simulink model "warplab_mimo_4x4"  (Simulink 6.5)
settings: Solver=ode45  StartTime=0.0  StopTime=20000  RelTol=1e-3
undefined symbols (not defined in the file): gcbh, xlBlockLoadCallback
libraries: xbsIndex_r4 x188
(part 14 of 17)

== system warplab_mimo_4x4/Radio_3_Inputs/ADC_I ==
  Constant1 : Constant  Value=0  OutDataType=sfix(16)  ConRadixGroup=Use specified scaling  OutScaling=2^0  SampleTime=inf  FramePeriod=inf
  Radio_3_ADC_I : Subsystem  mask{adc_sample_period=1}
      mask prompts: adc_sample_period "Sample Period"
      mask Display: image(imread('WARP_Logo.jpg'))
  Register : S-Function  LoadFcn=xlBlockLoadCallback(gcbh);  FunctionName=sysgen  Parameters=ptable_  mask(Xilinx Register Block){init=0, rst_sgadvanced=, rst=off, en_sgadvanced=, en=off, dbl_ovrd_sgadvanced=, dbl_ovrd=off, xl_use_area_sgadvanced=, xl_use_area=off, xl_area=[0,0,0,0,0,0,0], has_advanced_control=0, sggui_pos=-1,-1,-1,-1, block_type=register, block_version=8.2, sg_icon_stat=35,28,1,1,white,blue,0,ac6b57db, sg_mask_display=|, sg_list_contents=, sg_blockgui_xml=}
      mask sg_mask_display=|
      | fprintf('','COMMENT: begin icon graphics');
      | patch([0 35 35 0 ],[0 0 28 28 ],[0.77 0.82 0.91]);
      | patch([10 5 12 5 10 17 19 21 29 23 17 13 21 13 17 23 29 21 19 17 10 ],[3 8 15 22 27 27 25 27 27 21 27 23 15 7 3 9 3 3 5 3 3 ],[0.98 0.96 0.92]);
      | plot([0 0 35 35 0 ],[0 28 28 0 0 ]);
      | fprintf('','COMMENT: end icon graphics');
      | fprintf('','COMMENT: begin icon text');
      | color('black');port_label('input',1,'d');
      | color('black');port_label('output',1,'q');
      | color('black');disp('\bf{z^{-1}}','texmode','on');
      | fprintf('','COMMENT: end icon text');
      mask prompts: init "Initial value"; rst_sgadvanced ""; rst "Provide synchronous reset port"; en_sgadvanced ""; en "Provide enable port"; dbl_ovrd_sgadvanced ""; dbl_ovrd "Override with doubles"; xl_use_area_sgadvanced ""; xl_use_area "Define FPGA area for resource estimation"; xl_area "FPGA area [slices, FFs, BRAMs, LUTs, IOBs, emb. mults, TBUFs]"; has_advanced_control ""; sggui_pos ""; block_type ""; block_version ""; sg_icon_stat ""; sg_mask_display ""; sg_list_contents ""; sg_blockgui_xml ""
      mask help: Xilinx Register
      mask init: same as warplab_mimo_4x4/Mem_Control/Register
      settings: CopyFcn=xlBlockMoveCallback(gcbh);  DeleteFcn=xlDestroyGui(gcbh);  ModelCloseFcn=xlDestroyGui(gcbh);  PreSaveFcn=xlBlockPreSaveCallback(gcbh);  PostSaveFcn=xlBlockPostSaveCallback(gcbh);  DestroyFcn=xlDestroyGui(gcbh);  OpenFcn=xlOpenGui(gcbh, 'register_gui.xml', @xlmagicenablement, -1)  CloseFcn=xlDestroyGui(gcbh);  MoveFcn=xlBlockMoveCallback(gcbh);
      mask Help: eval('xlWeb(xlhtmldoclink(''Register''))');
      mask Display:
      | fprintf('','COMMENT: begin icon graphics');
      | patch([0 35 35 0 ],[0 0 28 28 ],[0.77 0.82 0.91]);
      | patch([10 5 12 5 10 17 19 21 29 23 17 13 21 13 17 23 29 21 19 17 10 ],[3 8 15 22 27 27 25 27 27 21 27 23 15 7 3 9 3 3 5 3 3 ],[0.98 0.96 0.92]);
      | plot([0 0 35 35 0 ],[0 28 28 0 0 ]);
      | fprintf('','COMMENT: end icon graphics');
      | fprintf('','COMMENT: begin icon text');
      | color('black');port_label('input',1,'d');
      | color('black');port_label('output',1,'q');
      | color('black');disp('\bf{z^{-1}}','texmode','on');
      | fprintf('','COMMENT: end icon text');
  radio3_ADC_I_OTR : S-Function  LoadFcn=xlBlockLoadCallback(gcbh);  FunctionName=sysgen  Parameters=ptable_  mask(Xilinx Gateway In Block){infoedit=Gateway in block.  Converts inputs of type Simulink integer, double and fixed point to  Xilinx fixed point type.<P><P>Hardware notes:  In hardware these blocks become top level input ports., arith_type_sgadvanced=, arith_type=Unsigned, n_bits=1, bin_pt=0, quantization_sgadvanced=, quantization=Round  (unbiased: +/- Inf), overflow_sgadvanced=, overflow=Saturate, period=1, dbl_ovrd_sgadvanced=, dbl_ovrd=off, timing_constraint_sgadvanced=, timing_constraint=None, locs_specified_sgadvanced=, locs_specified=off, LOCs={}, xl_use_area_sgadvanced=, xl_use_area=off, xl_area=[0,0,0,0,0,0,0], sginterface=, has_advanced_control=0, sggui_pos=20,20,356,432, block_type=gatewayin, block_version=VER_STRING_GOES_HERE, sg_icon_stat=55,12,1,1,white,yellow,0,4bb76ffd, sg_mask_display=|, sg_list_contents=, sg_blockgui_xml=}
      mask sg_mask_display=|
      | fprintf('','COMMENT: begin icon graphics ');
      | patch([0 55 55 0 ],[0 0 12 12 ],[0.95 0.93 0.65]);
      | patch([24 22 25 22 24 27 28 29 32 29 26 24 27 24 26 29 32 29 28 27 24 ],[1 3 6 9 11 11 10 11 11 8 11 9 6 3 1 4 1 1 2 1 1 ],[0.98 0.96 0.92]);
      | plot([0 0 55 55 0 ],[0 12 12 0 0 ]);
      | fprintf('','COMMENT: end icon graphics');
      |
      | fprintf('','COMMENT: begin icon text ');
      | color('black');port_label('input',1,'\fontsize{11pt}\bf In ','texmode','on');
      | color('black');port_label('output',1,' ');
      | fprintf('','COMMENT: end icon text');
      | fprintf('','COMMENT: Make no changes above this line -- machine generated code. ');
      mask prompts: infoedit ""; arith_type_sgadvanced ""; arith_type "Output type"; n_bits "Number of bits"; bin_pt "Binary point"; quantization_sgadvanced ""; overflow_sgadvanced ""; period "Sample period"; dbl_ovrd_sgadvanced ""; dbl_ovrd "Override with doubles"; timing_constraint_sgadvanced ""; timing_constraint "IOB timing constraint"; locs_specified_sgadvanced ""; locs_specified "Specify IOB location constraints"; LOCs "IOB pad locations (specify as cell array {'MSB', ..., 'LSB'})"; xl_use_area_sgadvanced ""; xl_use_area "Define FPGA area for resource estimation"; xl_area "FPGA area [slices, FFs, BRAMs, LUTs, IOBs, emb. mults, TBUFs]"; sginterface ""; has_advanced_control ""; sggui_pos ""; block_type ""; block_version ""; sg_icon_stat ""; sg_mask_display ""; sg_list_contents ""; sg_blockgui_xml ""
      mask help:
      | Gateway in block.  Converts inputs of type Simulink integer, double and fixed point to  Xilinx fixed point type.
      |
      | Hardware notes:  In hardware these blocks become top level input ports.
      mask init: same as warplab_mimo_4x4/StartCapture
      settings: CopyFcn=xlBlockMoveCallback(gcbh);  DeleteFcn=xlDestroyGui(gcbh);  ModelCloseFcn=xlDestroyGui(gcbh);  PreSaveFcn=xlBlockPreSaveCallback(gcbh);  PostSaveFcn=xlBlockPostSaveCallback(gcbh);  DestroyFcn=xlDestroyGui(gcbh);  OpenFcn=xlOpenGui(gcbh, 'gatewayin_gui.xml', @gatewayinenablement, @gatewayinaction)  CloseFcn=xlDestroyGui(gcbh);  MoveFcn=xlBlockMoveCallback(gcbh);
      mask Help: eval('xlWeb(xlhtmldoclink(''Gateway In''))');
      mask StyleString: edit,edit,popup(Boolean|Signed  (2's comp)|Unsigned),edit,edit,edit,popup(Truncate|Round  (unbiased: +/- Inf)),edit,popup(Wrap|Saturate|Flag as error),edit,edit,checkbox,edit,popup(None|Data Rate),edit,checkbox,edit,edit,checkbox,edit,edit,edit,edit,edit,edit,edit,edit,edit,edit
      mask Display:
      | fprintf('','COMMENT: begin icon graphics ');
      | patch([0 55 55 0 ],[0 0 12 12 ],[0.95 0.93 0.65]);
      | patch([24 22 25 22 24 27 28 29 32 29 26 24 27 24 26 29 32 29 28 27 24 ],[1 3 6 9 11 11 10 11 11 8 11 9 6 3 1 4 1 1 2 1 1 ],[0.98 0.96 0.92]);
      | plot([0 0 55 55 0 ],[0 12 12 0 0 ]);
      | fprintf('','COMMENT: end icon graphics');
      | 
      | fprintf('','COMMENT: begin icon text ');
      | color('black');port_label('input',1,'\fontsize{11pt}\bf In ','texmode','on');
      | color('black');port_label('output',1,' ');
      | fprintf('','COMMENT: end icon text');
      | fprintf('','COMMENT: Make no changes above this line -- machine generated code. ');
  OTR I : Outport
  ADC I : Outport  Port=2
  wires:
  Register/1 -> ADC I/1
  radio3_ADC_I_OTR/1 -> OTR I/1
  Radio_3_ADC_I/1(I_out) -> Register/1
  Constant1/1 -> radio3_ADC_I_OTR/1, Radio_3_ADC_I/1(I)

== system warplab_mimo_4x4/Radio_3_Inputs/ADC_Q ==
  Constant1 : Constant  Value=0  OutDataType=sfix(16)  ConRadixGroup=Use specified scaling  OutScaling=2^0  SampleTime=inf  FramePeriod=inf
  Radio_3_ADC_Q : Subsystem  mask{adc_sample_period=1}
      mask Display: image(imread('WARP_Logo.jpg'))
  Register : S-Function  LoadFcn=xlBlockLoadCallback(gcbh);  FunctionName=sysgen  Parameters=ptable_  mask(Xilinx Register Block){init=0, rst_sgadvanced=, rst=off, en_sgadvanced=, en=off, dbl_ovrd_sgadvanced=, dbl_ovrd=off, xl_use_area_sgadvanced=, xl_use_area=off, xl_area=[0,0,0,0,0,0,0], has_advanced_control=0, sggui_pos=-1,-1,-1,-1, block_type=register, block_version=8.2, sg_icon_stat=35,28,1,1,white,blue,0,ac6b57db, sg_mask_display=|, sg_list_contents=, sg_blockgui_xml=}
      mask sg_mask_display=|
      | fprintf('','COMMENT: begin icon graphics');
      | patch([0 35 35 0 ],[0 0 28 28 ],[0.77 0.82 0.91]);
      | patch([10 5 12 5 10 17 19 21 29 23 17 13 21 13 17 23 29 21 19 17 10 ],[3 8 15 22 27 27 25 27 27 21 27 23 15 7 3 9 3 3 5 3 3 ],[0.98 0.96 0.92]);
      | plot([0 0 35 35 0 ],[0 28 28 0 0 ]);
      | fprintf('','COMMENT: end icon graphics');
      | fprintf('','COMMENT: begin icon text');
      | color('black');port_label('input',1,'d');
      | color('black');port_label('output',1,'q');
      | color('black');disp('\bf{z^{-1}}','texmode','on');
      | fprintf('','COMMENT: end icon text');
      mask prompts: init "Initial value"; rst_sgadvanced ""; rst "Provide synchronous reset port"; en_sgadvanced ""; en "Provide enable port"; dbl_ovrd_sgadvanced ""; dbl_ovrd "Override with doubles"; xl_use_area_sgadvanced ""; xl_use_area "Define FPGA area for resource estimation"; xl_area "FPGA area [slices, FFs, BRAMs, LUTs, IOBs, emb. mults, TBUFs]"; has_advanced_control ""; sggui_pos ""; block_type ""; block_version ""; sg_icon_stat ""; sg_mask_display ""; sg_list_contents ""; sg_blockgui_xml ""
      mask help: Xilinx Register
      mask init: same as warplab_mimo_4x4/Mem_Control/Register
      settings: CopyFcn=xlBlockMoveCallback(gcbh);  DeleteFcn=xlDestroyGui(gcbh);  ModelCloseFcn=xlDestroyGui(gcbh);  PreSaveFcn=xlBlockPreSaveCallback(gcbh);  PostSaveFcn=xlBlockPostSaveCallback(gcbh);  DestroyFcn=xlDestroyGui(gcbh);  OpenFcn=xlOpenGui(gcbh, 'register_gui.xml', @xlmagicenablement, -1)  CloseFcn=xlDestroyGui(gcbh);  MoveFcn=xlBlockMoveCallback(gcbh);
      mask Help: eval('xlWeb(xlhtmldoclink(''Register''))');
      mask Display:
      | fprintf('','COMMENT: begin icon graphics');
      | patch([0 35 35 0 ],[0 0 28 28 ],[0.77 0.82 0.91]);
      | patch([10 5 12 5 10 17 19 21 29 23 17 13 21 13 17 23 29 21 19 17 10 ],[3 8 15 22 27 27 25 27 27 21 27 23 15 7 3 9 3 3 5 3 3 ],[0.98 0.96 0.92]);
      | plot([0 0 35 35 0 ],[0 28 28 0 0 ]);
      | fprintf('','COMMENT: end icon graphics');
      | fprintf('','COMMENT: begin icon text');
      | color('black');port_label('input',1,'d');
      | color('black');port_label('output',1,'q');
      | color('black');disp('\bf{z^{-1}}','texmode','on');
      | fprintf('','COMMENT: end icon text');
  radio3_ADC_Q_OTR : S-Function  LoadFcn=xlBlockLoadCallback(gcbh);  FunctionName=sysgen  Parameters=ptable_  mask(Xilinx Gateway In Block){infoedit=Gateway in block.  Converts inputs of type Simulink integer, double and fixed point to  Xilinx fixed point type.<P><P>Hardware notes:  In hardware these blocks become top level input ports., arith_type_sgadvanced=, arith_type=Unsigned, n_bits=1, bin_pt=0, quantization_sgadvanced=, quantization=Round  (unbiased: +/- Inf), overflow_sgadvanced=, overflow=Saturate, period=1, dbl_ovrd_sgadvanced=, dbl_ovrd=off, timing_constraint_sgadvanced=, timing_constraint=None, locs_specified_sgadvanced=, locs_specified=off, LOCs={}, xl_use_area_sgadvanced=, xl_use_area=off, xl_area=[0,0,0,0,0,0,0], sginterface=, has_advanced_control=0, sggui_pos=20,20,356,432, block_type=gatewayin, block_version=VER_STRING_GOES_HERE, sg_icon_stat=55,12,1,1,white,yellow,0,4bb76ffd, sg_mask_display=|, sg_list_contents=, sg_blockgui_xml=}
      mask sg_mask_display=|
      | fprintf('','COMMENT: begin icon graphics ');
      | patch([0 55 55 0 ],[0 0 12 12 ],[0.95 0.93 0.65]);
      | patch([24 22 25 22 24 27 28 29 32 29 26 24 27 24 26 29 32 29 28 27 24 ],[1 3 6 9 11 11 10 11 11 8 11 9 6 3 1 4 1 1 2 1 1 ],[0.98 0.96 0.92]);
      | plot([0 0 55 55 0 ],[0 12 12 0 0 ]);
      | fprintf('','COMMENT: end icon graphics');
      |
      | fprintf('','COMMENT: begin icon text ');
      | color('black');port_label('input',1,'\fontsize{11pt}\bf In ','texmode','on');
      | color('black');port_label('output',1,' ');
      | fprintf('','COMMENT: end icon text');
      | fprintf('','COMMENT: Make no changes above this line -- machine generated code. ');
      mask prompts: infoedit ""; arith_type_sgadvanced ""; arith_type "Output type"; n_bits "Number of bits"; bin_pt "Binary point"; quantization_sgadvanced ""; overflow_sgadvanced ""; period "Sample period"; dbl_ovrd_sgadvanced ""; dbl_ovrd "Override with doubles"; timing_constraint_sgadvanced ""; timing_constraint "IOB timing constraint"; locs_specified_sgadvanced ""; locs_specified "Specify IOB location constraints"; LOCs "IOB pad locations (specify as cell array {'MSB', ..., 'LSB'})"; xl_use_area_sgadvanced ""; xl_use_area "Define FPGA area for resource estimation"; xl_area "FPGA area [slices, FFs, BRAMs, LUTs, IOBs, emb. mults, TBUFs]"; sginterface ""; has_advanced_control ""; sggui_pos ""; block_type ""; block_version ""; sg_icon_stat ""; sg_mask_display ""; sg_list_contents ""; sg_blockgui_xml ""
      mask help:
      | Gateway in block.  Converts inputs of type Simulink integer, double and fixed point to  Xilinx fixed point type.
      |
      | Hardware notes:  In hardware these blocks become top level input ports.
      mask init: same as warplab_mimo_4x4/StartCapture
      settings: CopyFcn=xlBlockMoveCallback(gcbh);  DeleteFcn=xlDestroyGui(gcbh);  ModelCloseFcn=xlDestroyGui(gcbh);  PreSaveFcn=xlBlockPreSaveCallback(gcbh);  PostSaveFcn=xlBlockPostSaveCallback(gcbh);  DestroyFcn=xlDestroyGui(gcbh);  OpenFcn=xlOpenGui(gcbh, 'gatewayin_gui.xml', @gatewayinenablement, @gatewayinaction)  CloseFcn=xlDestroyGui(gcbh);  MoveFcn=xlBlockMoveCallback(gcbh);
      mask Help: eval('xlWeb(xlhtmldoclink(''Gateway In''))');
      mask StyleString: edit,edit,popup(Boolean|Signed  (2's comp)|Unsigned),edit,edit,edit,popup(Truncate|Round  (unbiased: +/- Inf)),edit,popup(Wrap|Saturate|Flag as error),edit,edit,checkbox,edit,popup(None|Data Rate),edit,checkbox,edit,edit,checkbox,edit,edit,edit,edit,edit,edit,edit,edit,edit,edit
      mask Display:
      | fprintf('','COMMENT: begin icon graphics ');
      | patch([0 55 55 0 ],[0 0 12 12 ],[0.95 0.93 0.65]);
      | patch([24 22 25 22 24 27 28 29 32 29 26 24 27 24 26 29 32 29 28 27 24 ],[1 3 6 9 11 11 10 11 11 8 11 9 6 3 1 4 1 1 2 1 1 ],[0.98 0.96 0.92]);
      | plot([0 0 55 55 0 ],[0 12 12 0 0 ]);
      | fprintf('','COMMENT: end icon graphics');
      | 
      | fprintf('','COMMENT: begin icon text ');
      | color('black');port_label('input',1,'\fontsize{11pt}\bf In ','texmode','on');
      | color('black');port_label('output',1,' ');
      | fprintf('','COMMENT: end icon text');
      | fprintf('','COMMENT: Make no changes above this line -- machine generated code. ');
  OTR Q : Outport
  ADC Q : Outport  Port=2
  wires:
  Register/1 -> ADC Q/1
  Constant1/1 -> radio3_ADC_Q_OTR/1, Radio_3_ADC_Q/1(Q)
  Radio_3_ADC_Q/1(Q_out) -> Register/1
  radio3_ADC_Q_OTR/1 -> OTR Q/1

== system warplab_mimo_4x4/Radio_3_Inputs/Concatenates_1 ==
  OTR_I : Inport
  ADC_I : Inport  Port=2
  OTR_Q : Inport  Port=3
  ADC_Q : Inport  Port=4
  Concat1 : S-Function  LoadFcn=xlBlockLoadCallback(gcbh);  FunctionName=sysgen  Parameters=ptable_  mask(Xilinx Bus Concatenator Block){infoedit=Concatenates two or more inputs.  Output will be cast to an unsigned value with the binary point at zero., num_inputs=2, dbl_ovrd_sgadvanced=, dbl_ovrd=off, has_advanced_control=0, sggui_pos=-1,-1,-1,-1, block_type=concat, block_version=8.2, sg_icon_stat=30,38,2,1,white,blue,0,59d62d82, sg_mask_display=|, sg_list_contents=, sg_blockgui_xml=}
      mask sg_mask_display=|
      | fprintf('','COMMENT: begin icon graphics');
      | patch([0 30 30 0 ],[0 0 38 38 ],[0.77 0.82 0.91]);
      | patch([7 2 9 2 7 15 17 19 27 20 14 9 15 9 14 20 27 19 17 15 7 ],[7 12 19 26 31 31 29 31 31 24 30 25 19 13 8 14 7 7 9 7 7 ],[0.98 0.96 0.92]);
      | plot([0 0 30 30 0 ],[0 38 38 0 0 ]);
      | fprintf('','COMMENT: end icon graphics');
      | fprintf('','COMMENT: begin icon text');
      | color('black');port_label('input',1,'hi');
      | color('black');port_label('input',2,'lo');
      | fprintf('','COMMENT: end icon text');
      mask prompts: infoedit ""; num_inputs "Number of inputs"; dbl_ovrd_sgadvanced ""; dbl_ovrd "Override with doubles"; has_advanced_control ""; sggui_pos ""; block_type ""; block_version ""; sg_icon_stat ""; sg_mask_display ""; sg_list_contents ""; sg_blockgui_xml ""
      mask help: Concatenates two or more inputs. Output will be cast to an unsigned value with the binary point at zero.
      mask init: same as warplab_mimo_4x4/Radio_1_Inputs/Concatenates_1/Concat1
      settings: CopyFcn=xlBlockMoveCallback(gcbh);  DeleteFcn=xlDestroyGui(gcbh);  ModelCloseFcn=xlDestroyGui(gcbh);  PreSaveFcn=xlBlockPreSaveCallback(gcbh);  PostSaveFcn=xlBlockPostSaveCallback(gcbh);  DestroyFcn=xlDestroyGui(gcbh);  OpenFcn=xlOpenGui(gcbh, 'concat_gui.xml', @xlmagicenablement, -1)  CloseFcn=xlDestroyGui(gcbh);  MoveFcn=xlBlockMoveCallback(gcbh);
      mask Help: eval('xlWeb(xlhtmldoclink(''Concat''))');
      mask Display:
      | fprintf('','COMMENT: begin icon graphics');
      | patch([0 30 30 0 ],[0 0 38 38 ],[0.77 0.82 0.91]);
      | patch([7 2 9 2 7 15 17 19 27 20 14 9 15 9 14 20 27 19 17 15 7 ],[7 12 19 26 31 31 29 31 31 24 30 25 19 13 8 14 7 7 9 7 7 ],[0.98 0.96 0.92]);
      | plot([0 0 30 30 0 ],[0 38 38 0 0 ]);
      | fprintf('','COMMENT: end icon graphics');
      | fprintf('','COMMENT: begin icon text');
      | color('black');port_label('input',1,'hi');
      | color('black');port_label('input',2,'lo');
      | fprintf('','COMMENT: end icon text');
  Concat2 : S-Function  LoadFcn=xlBlockLoadCallback(gcbh);  FunctionName=sysgen  Parameters=ptable_  mask(Xilinx Bus Concatenator Block){infoedit=Concatenates two or more inputs.  Output will be cast to an unsigned value with the binary point at zero., num_inputs=2, dbl_ovrd_sgadvanced=, dbl_ovrd=off, has_advanced_control=0, sggui_pos=-1,-1,-1,-1, block_type=concat, block_version=8.2, sg_icon_stat=30,38,2,1,white,blue,0,59d62d82, sg_mask_display=|, sg_list_contents=, sg_blockgui_xml=}
      mask sg_mask_display=|
      | fprintf('','COMMENT: begin icon graphics');
      | patch([0 30 30 0 ],[0 0 38 38 ],[0.77 0.82 0.91]);
      | patch([7 2 9 2 7 15 17 19 27 20 14 9 15 9 14 20 27 19 17 15 7 ],[7 12 19 26 31 31 29 31 31 24 30 25 19 13 8 14 7 7 9 7 7 ],[0.98 0.96 0.92]);
      | plot([0 0 30 30 0 ],[0 38 38 0 0 ]);
      | fprintf('','COMMENT: end icon graphics');
      | fprintf('','COMMENT: begin icon text');
      | color('black');port_label('input',1,'hi');
      | color('black');port_label('input',2,'lo');
      | fprintf('','COMMENT: end icon text');
      mask prompts: infoedit ""; num_inputs "Number of inputs"; dbl_ovrd_sgadvanced ""; dbl_ovrd "Override with doubles"; has_advanced_control ""; sggui_pos ""; block_type ""; block_version ""; sg_icon_stat ""; sg_mask_display ""; sg_list_contents ""; sg_blockgui_xml ""
      mask help: Concatenates two or more inputs. Output will be cast to an unsigned value with the binary point at zero.
      mask init: same as warplab_mimo_4x4/Radio_1_Inputs/Concatenates_1/Concat1
      settings: CopyFcn=xlBlockMoveCallback(gcbh);  DeleteFcn=xlDestroyGui(gcbh);  ModelCloseFcn=xlDestroyGui(gcbh);  PreSaveFcn=xlBlockPreSaveCallback(gcbh);  PostSaveFcn=xlBlockPostSaveCallback(gcbh);  DestroyFcn=xlDestroyGui(gcbh);  OpenFcn=xlOpenGui(gcbh, 'concat_gui.xml', @xlmagicenablement, -1)  CloseFcn=xlDestroyGui(gcbh);  MoveFcn=xlBlockMoveCallback(gcbh);
      mask Help: eval('xlWeb(xlhtmldoclink(''Concat''))');
      mask Display:
      | fprintf('','COMMENT: begin icon graphics');
      | patch([0 30 30 0 ],[0 0 38 38 ],[0.77 0.82 0.91]);
      | patch([7 2 9 2 7 15 17 19 27 20 14 9 15 9 14 20 27 19 17 15 7 ],[7 12 19 26 31 31 29 31 31 24 30 25 19 13 8 14 7 7 9 7 7 ],[0.98 0.96 0.92]);
      | plot([0 0 30 30 0 ],[0 38 38 0 0 ]);
      | fprintf('','COMMENT: end icon graphics');
      | fprintf('','COMMENT: begin icon text');
      | color('black');port_label('input',1,'hi');
      | color('black');port_label('input',2,'lo');
      | fprintf('','COMMENT: end icon text');
  Concat3 : S-Function  LoadFcn=xlBlockLoadCallback(gcbh);  FunctionName=sysgen  Parameters=ptable_  mask(Xilinx Bus Concatenator Block){infoedit=Concatenates two or more inputs.  Output will be cast to an unsigned value with the binary point at zero., num_inputs=2, dbl_ovrd_sgadvanced=, dbl_ovrd=off, has_advanced_control=0, sggui_pos=-1,-1,-1,-1, block_type=concat, block_version=8.2, sg_icon_stat=25,80,2,1,white,blue,0,59d62d82, sg_mask_display=|, sg_list_contents=, sg_blockgui_xml=}
      mask sg_mask_display=|
      | fprintf('','COMMENT: begin icon graphics');
      | patch([0 25 25 0 ],[0 0 80 80 ],[0.77 0.82 0.91]);
      | patch([6 2 8 2 6 13 15 17 24 18 13 9 14 9 13 18 24 17 15 13 6 ],[30 34 40 46 50 50 48 50 50 44 49 45 40 35 31 36 30 30 32 30 30 ],[0.98 0.96 0.92]);
      | plot([0 0 25 25 0 ],[0 80 80 0 0 ]);
      | fprintf('','COMMENT: end icon graphics');
      | fprintf('','COMMENT: begin icon text');
      | color('black');port_label('input',1,'hi');
      | color('black');port_label('input',2,'lo');
      | fprintf('','COMMENT: end icon text');
      mask prompts: infoedit ""; num_inputs "Number of inputs"; dbl_ovrd_sgadvanced ""; dbl_ovrd "Override with doubles"; has_advanced_control ""; sggui_pos ""; block_type ""; block_version ""; sg_icon_stat ""; sg_mask_display ""; sg_list_contents ""; sg_blockgui_xml ""
      mask help: Concatenates two or more inputs. Output will be cast to an unsigned value with the binary point at zero.
      mask init: same as warplab_mimo_4x4/Radio_1_Inputs/Concatenates_1/Concat1
      settings: CopyFcn=xlBlockMoveCallback(gcbh);  DeleteFcn=xlDestroyGui(gcbh);  ModelCloseFcn=xlDestroyGui(gcbh);  PreSaveFcn=xlBlockPreSaveCallback(gcbh);  PostSaveFcn=xlBlockPostSaveCallback(gcbh);  DestroyFcn=xlDestroyGui(gcbh);  OpenFcn=xlOpenGui(gcbh, 'concat_gui.xml', @xlmagicenablement, -1)  CloseFcn=xlDestroyGui(gcbh);  MoveFcn=xlBlockMoveCallback(gcbh);
      mask Help: eval('xlWeb(xlhtmldoclink(''Concat''))');
      mask Display:
      | fprintf('','COMMENT: begin icon graphics');
      | patch([0 25 25 0 ],[0 0 80 80 ],[0.77 0.82 0.91]);
      | patch([6 2 8 2 6 13 15 17 24 18 13 9 14 9 13 18 24 17 15 13 6 ],[30 34 40 46 50 50 48 50 50 44 49 45 40 35 31 36 30 30 32 30 30 ],[0.98 0.96 0.92]);
      | plot([0 0 25 25 0 ],[0 80 80 0 0 ]);
      | fprintf('','COMMENT: end icon graphics');
      | fprintf('','COMMENT: begin icon text');
      | color('black');port_label('input',1,'hi');
      | color('black');port_label('input',2,'lo');
      | fprintf('','COMMENT: end icon text');
  Concat4 : S-Function  LoadFcn=xlBlockLoadCallback(gcbh);  FunctionName=sysgen  Parameters=ptable_  mask(Xilinx Bus Concatenator Block){infoedit=Concatenates two or more inputs.  Output will be cast to an unsigned value with the binary point at zero., num_inputs=2, dbl_ovrd_sgadvanced=, dbl_ovrd=off, has_advanced_control=0, sggui_pos=-1,-1,-1,-1, block_type=concat, block_version=8.2, sg_icon_stat=25,80,2,1,white,blue,0,59d62d82, sg_mask_display=|, sg_list_contents=, sg_blockgui_xml=}
      mask sg_mask_display=|
      | fprintf('','COMMENT: begin icon graphics');
      | patch([0 25 25 0 ],[0 0 80 80 ],[0.77 0.82 0.91]);
      | patch([6 2 8 2 6 13 15 17 24 18 13 9 14 9 13 18 24 17 15 13 6 ],[30 34 40 46 50 50 48 50 50 44 49 45 40 35 31 36 30 30 32 30 30 ],[0.98 0.96 0.92]);
      | plot([0 0 25 25 0 ],[0 80 80 0 0 ]);
      | fprintf('','COMMENT: end icon graphics');
      | fprintf('','COMMENT: begin icon text');
      | color('black');port_label('input',1,'hi');
      | color('black');port_label('input',2,'lo');
      | fprintf('','COMMENT: end icon text');
      mask prompts: infoedit ""; num_inputs "Number of inputs"; dbl_ovrd_sgadvanced ""; dbl_ovrd "Override with doubles"; has_advanced_control ""; sggui_pos ""; block_type ""; block_version ""; sg_icon_stat ""; sg_mask_display ""; sg_list_contents ""; sg_blockgui_xml ""
      mask help: Concatenates two or more inputs. Output will be cast to an unsigned value with the binary point at zero.
      mask init: same as warplab_mimo_4x4/Radio_1_Inputs/Concatenates_1/Concat1
      settings: CopyFcn=xlBlockMoveCallback(gcbh);  DeleteFcn=xlDestroyGui(gcbh);  ModelCloseFcn=xlDestroyGui(gcbh);  PreSaveFcn=xlBlockPreSaveCallback(gcbh);  PostSaveFcn=xlBlockPostSaveCallback(gcbh);  DestroyFcn=xlDestroyGui(gcbh);  OpenFcn=xlOpenGui(gcbh, 'concat_gui.xml', @xlmagicenablement, -1)  CloseFcn=xlDestroyGui(gcbh);  MoveFcn=xlBlockMoveCallback(gcbh);
      mask Help: eval('xlWeb(xlhtmldoclink(''Concat''))');
      mask Display:
      | fprintf('','COMMENT: begin icon graphics');
      | patch([0 25 25 0 ],[0 0 80 80 ],[0.77 0.82 0.91]);
      | patch([6 2 8 2 6 13 15 17 24 18 13 9 14 9 13 18 24 17 15 13 6 ],[30 34 40 46 50 50 48 50 50 44 49 45 40 35 31 36 30 30 32 30 30 ],[0.98 0.96 0.92]);
      | plot([0 0 25 25 0 ],[0 80 80 0 0 ]);
      | fprintf('','COMMENT: end icon graphics');
      | fprintf('','COMMENT: begin icon text');
      | color('black');port_label('input',1,'hi');
      | color('black');port_label('input',2,'lo');
      | fprintf('','COMMENT: end icon text');
  Concat5 : S-Function  LoadFcn=xlBlockLoadCallback(gcbh);  FunctionName=sysgen  Parameters=ptable_  mask(Xilinx Bus Concatenator Block){infoedit=Concatenates two or more inputs.  Output will be cast to an unsigned value with the binary point at zero., num_inputs=2, dbl_ovrd_sgadvanced=, dbl_ovrd=off, has_advanced_control=0, sggui_pos=-1,-1,-1,-1, block_type=concat, block_version=8.2, sg_icon_stat=25,80,2,1,white,blue,0,59d62d82, sg_mask_display=|, sg_list_contents=, sg_blockgui_xml=}
      mask sg_mask_display=|
      | fprintf('','COMMENT: begin icon graphics');
      | patch([0 25 25 0 ],[0 0 80 80 ],[0.77 0.82 0.91]);
      | patch([6 2 8 2 6 13 15 17 24 18 13 9 14 9 13 18 24 17 15 13 6 ],[30 34 40 46 50 50 48 50 50 44 49 45 40 35 31 36 30 30 32 30 30 ],[0.98 0.96 0.92]);
      | plot([0 0 25 25 0 ],[0 80 80 0 0 ]);
      | fprintf('','COMMENT: end icon graphics');
      | fprintf('','COMMENT: begin icon text');
      | color('black');port_label('input',1,'hi');
      | color('black');port_label('input',2,'lo');
      | fprintf('','COMMENT: end icon text');
      mask prompts: infoedit ""; num_inputs "Number of inputs"; dbl_ovrd_sgadvanced ""; dbl_ovrd "Override with doubles"; has_advanced_control ""; sggui_pos ""; block_type ""; block_version ""; sg_icon_stat ""; sg_mask_display ""; sg_list_contents ""; sg_blockgui_xml ""
      mask help: Concatenates two or more inputs. Output will be cast to an unsigned value with the binary point at zero.
      mask init: same as warplab_mimo_4x4/Radio_1_Inputs/Concatenates_1/Concat1
      settings: CopyFcn=xlBlockMoveCallback(gcbh);  DeleteFcn=xlDestroyGui(gcbh);  ModelCloseFcn=xlDestroyGui(gcbh);  PreSaveFcn=xlBlockPreSaveCallback(gcbh);  PostSaveFcn=xlBlockPostSaveCallback(gcbh);  DestroyFcn=xlDestroyGui(gcbh);  OpenFcn=xlOpenGui(gcbh, 'concat_gui.xml', @xlmagicenablement, -1)  CloseFcn=xlDestroyGui(gcbh);  MoveFcn=xlBlockMoveCallback(gcbh);
      mask Help: eval('xlWeb(xlhtmldoclink(''Concat''))');
      mask Display:
      | fprintf('','COMMENT: begin icon graphics');
      | patch([0 25 25 0 ],[0 0 80 80 ],[0.77 0.82 0.91]);
      | patch([6 2 8 2 6 13 15 17 24 18 13 9 14 9 13 18 24 17 15 13 6 ],[30 34 40 46 50 50 48 50 50 44 49 45 40 35 31 36 30 30 32 30 30 ],[0.98 0.96 0.92]);
      | plot([0 0 25 25 0 ],[0 80 80 0 0 ]);
      | fprintf('','COMMENT: end icon graphics');
      | fprintf('','COMMENT: begin icon text');
      | color('black');port_label('input',1,'hi');
      | color('black');port_label('input',2,'lo');
      | fprintf('','COMMENT: end icon text');
  Reinterpret : S-Function  LoadFcn=xlBlockLoadCallback(gcbh);  FunctionName=sysgen  Parameters=ptable_  mask(Xilinx Type Reinterpreter Block){infoedit=Changes signal type without altering the binary representation.   You can changed the signal between signed and unsigned, and relocate the binary point.<P><P>Hardware notes: In hardware this block costs nothing.<P><P>Example:  Suppose the input is 6 bits wide, signed, with 2 fractional bits, and the output is forced to unsigned with 0 fractional bits.  Then an input of -2.0 (1110.00 in binary 2's complement) becomes an output of 56 (111000 in binary)., force_arith_type_sgadvanced=, force_arith_type=on, arith_type_sgadvanced=, arith_type=Unsigned, force_bin_pt_sgadvanced=, force_bin_pt=on, bin_pt=0, has_advanced_control=0, sggui_pos=20,20,356,309, block_type=reinterpret, block_version=8.2, sg_icon_stat=35,20,1,1,white,blue,0,8982c1db, sg_mask_display=|, sg_list_contents=, sg_blockgui_xml=}
      mask sg_mask_display=|
      | fprintf('','COMMENT: begin icon graphics');
      | patch([0 35 35 0 ],[0 0 20 20 ],[0.77 0.82 0.91]);
      | patch([12 9 14 9 12 17 18 19 25 21 17 14 19 14 17 21 25 19 18 17 12 ],[2 5 10 15 18 18 17 18 18 14 18 15 10 5 2 6 2 2 3 2 2 ],[0.98 0.96 0.92]);
      | plot([0 0 35 35 0 ],[0 20 20 0 0 ]);
      | fprintf('','COMMENT: end icon graphics');
      | fprintf('','COMMENT: begin icon text');
      | color('black');disp('reinterpret');
      | fprintf('','COMMENT: end icon text');
      mask prompts: infoedit ""; force_arith_type_sgadvanced ""; force_arith_type "Force Arithmetic Type"; arith_type_sgadvanced ""; arith_type "Output Arithmetic Type"; force_bin_pt_sgadvanced ""; force_bin_pt "Force Binary Point"; bin_pt "Output Binary Point"; has_advanced_control ""; sggui_pos ""; block_type ""; block_version ""; sg_icon_stat ""; sg_mask_display ""; sg_list_contents ""; sg_blockgui_xml ""
      mask help:
      | Changes signal type without altering the binary representation.   You can changed the signal between signed and unsigned, and relocate the binary point.
      |
      | Hardware notes: In hardware this block costs nothing.
      |
      | Example:  Suppose the input is 6 bits wide, signed, with 2 fractional bits, and the output is forced to unsigned with 0 fractional bits.  Then an input of -2.0 (1110.00 in binary 2's complement) becomes an output of 56 (111000 in binary).
      mask init: same as warplab_mimo_4x4/Radio_1_Outputs/Reinterpret
      settings: CopyFcn=xlBlockMoveCallback(gcbh);  DeleteFcn=xlDestroyGui(gcbh);  ModelCloseFcn=xlDestroyGui(gcbh);  PreSaveFcn=xlBlockPreSaveCallback(gcbh);  PostSaveFcn=xlBlockPostSaveCallback(gcbh);  DestroyFcn=xlDestroyGui(gcbh);  OpenFcn=xlOpenGui(gcbh, 'reinterpret_gui.xml', @reinterpretenablement, -1)  CloseFcn=xlDestroyGui(gcbh);  MoveFcn=xlBlockMoveCallback(gcbh);
      mask Help: eval('xlWeb(xlhtmldoclink(''Reinterpret''))');
      mask StyleString: edit,edit,checkbox,edit,popup(Unsigned|Signed  (2's comp)),edit,checkbox,edit,edit,edit,edit,edit,edit,edit,edit,edit
      mask Display:
      | fprintf('','COMMENT: begin icon graphics');
      | patch([0 35 35 0 ],[0 0 20 20 ],[0.77 0.82 0.91]);
      | patch([12 9 14 9 12 17 18 19 25 21 17 14 19 14 17 21 25 19 18 17 12 ],[2 5 10 15 18 18 17 18 18 14 18 15 10 5 2 6 2 2 3 2 2 ],[0.98 0.96 0.92]);
      | plot([0 0 35 35 0 ],[0 20 20 0 0 ]);
      | fprintf('','COMMENT: end icon graphics');
      | fprintf('','COMMENT: begin icon text');
      | color('black');disp('reinterpret');
      | fprintf('','COMMENT: end icon text');
  Reinterpret1 : S-Function  LoadFcn=xlBlockLoadCallback(gcbh);  FunctionName=sysgen  Parameters=ptable_  mask(Xilinx Type Reinterpreter Block){infoedit=Changes signal type without altering the binary representation.   You can changed the signal between signed and unsigned, and relocate the binary point.<P><P>Hardware notes: In hardware this block costs nothing.<P><P>Example:  Suppose the input is 6 bits wide, signed, with 2 fractional bits, and the output is forced to unsigned with 0 fractional bits.  Then an input of -2.0 (1110.00 in binary 2's complement) becomes an output of 56 (111000 in binary)., force_arith_type_sgadvanced=, force_arith_type=on, arith_type_sgadvanced=, arith_type=Unsigned, force_bin_pt_sgadvanced=, force_bin_pt=on, bin_pt=0, has_advanced_control=0, sggui_pos=20,20,356,309, block_type=reinterpret, block_version=8.2, sg_icon_stat=35,20,1,1,white,blue,0,8982c1db, sg_mask_display=|, sg_list_contents=, sg_blockgui_xml=}
      mask sg_mask_display=|
      | fprintf('','COMMENT: begin icon graphics');
      | patch([0 35 35 0 ],[0 0 20 20 ],[0.77 0.82 0.91]);
      | patch([12 9 14 9 12 17 18 19 25 21 17 14 19 14 17 21 25 19 18 17 12 ],[2 5 10 15 18 18 17 18 18 14 18 15 10 5 2 6 2 2 3 2 2 ],[0.98 0.96 0.92]);
      | plot([0 0 35 35 0 ],[0 20 20 0 0 ]);
      | fprintf('','COMMENT: end icon graphics');
      | fprintf('','COMMENT: begin icon text');
      | color('black');disp('reinterpret');
      | fprintf('','COMMENT: end icon text');
      mask prompts: infoedit ""; force_arith_type_sgadvanced ""; force_arith_type "Force Arithmetic Type"; arith_type_sgadvanced ""; arith_type "Output Arithmetic Type"; force_bin_pt_sgadvanced ""; force_bin_pt "Force Binary Point"; bin_pt "Output Binary Point"; has_advanced_control ""; sggui_pos ""; block_type ""; block_version ""; sg_icon_stat ""; sg_mask_display ""; sg_list_contents ""; sg_blockgui_xml ""
      mask help:
      | Changes signal type without altering the binary representation.   You can changed the signal between signed and unsigned, and relocate the binary point.
      |
      | Hardware notes: In hardware this block costs nothing.
      |
      | Example:  Suppose the input is 6 bits wide, signed, with 2 fractional bits, and the output is forced to unsigned with 0 fractional bits.  Then an input of -2.0 (1110.00 in binary 2's complement) becomes an output of 56 (111000 in binary).
      mask init: same as warplab_mimo_4x4/Radio_1_Outputs/Reinterpret
      settings: CopyFcn=xlBlockMoveCallback(gcbh);  DeleteFcn=xlDestroyGui(gcbh);  ModelCloseFcn=xlDestroyGui(gcbh);  PreSaveFcn=xlBlockPreSaveCallback(gcbh);  PostSaveFcn=xlBlockPostSaveCallback(gcbh);  DestroyFcn=xlDestroyGui(gcbh);  OpenFcn=xlOpenGui(gcbh, 'reinterpret_gui.xml', @reinterpretenablement, -1)  CloseFcn=xlDestroyGui(gcbh);  MoveFcn=xlBlockMoveCallback(gcbh);
      mask Help: eval('xlWeb(xlhtmldoclink(''Reinterpret''))');
      mask StyleString: edit,edit,checkbox,edit,popup(Unsigned|Signed  (2's comp)),edit,checkbox,edit,edit,edit,edit,edit,edit,edit,edit,edit
      mask Display:
      | fprintf('','COMMENT: begin icon graphics');
      | patch([0 35 35 0 ],[0 0 20 20 ],[0.77 0.82 0.91]);
      | patch([12 9 14 9 12 17 18 19 25 21 17 14 19 14 17 21 25 19 18 17 12 ],[2 5 10 15 18 18 17 18 18 14 18 15 10 5 2 6 2 2 3 2 2 ],[0.98 0.96 0.92]);
      | plot([0 0 35 35 0 ],[0 20 20 0 0 ]);
      | fprintf('','COMMENT: end icon graphics');
      | fprintf('','COMMENT: begin icon text');
      | color('black');disp('reinterpret');
      | fprintf('','COMMENT: end icon text');
  zero : S-Function  LoadFcn=xlBlockLoadCallback(gcbh);  FunctionName=sysgen  Parameters=ptable_  mask(Xilinx Constant Block Block){arith_type_sgadvanced=, arith_type=Unsigned, const=0, n_bits=1, bin_pt=0, explicit_period_sgadvanced=, explicit_period=off, period=1, dsp48_infoedit=The use of this block for DSP48 instructions is deprecated.  Please use the Opmode block., equ=P=C, opselect_sgadvanced=, opselect=C, inp2_sgadvanced=, inp2=PCIN>>17, opr_sgadvanced=, opr=+, inp1_sgadvanced=, inp1=P, carry_sgadvanced=, carry=CIN, dbl_ovrd_sgadvanced=, dbl_ovrd=off, has_advanced_control=0, sggui_pos=-1,-1,-1,-1, block_type=constant, block_version=VER_STRING_GOES_HERE, sg_icon_stat=20,18,0,1,white,blue,0,c7c04a0c, sg_mask_display=|, sg_list_contents=, sg_blockgui_xml=}
      mask sg_mask_display=|
      | fprintf('','COMMENT: begin icon graphics');
      | patch([0 55 55 0 ],[0 0 26 26 ],[0.77 0.82 0.91]);
      | patch([20 16 22 16 20 27 29 31 38 32 26 22 28 22 26 32 38 31 29 27 20 ],[3 7 13 19 23 23 21 23 23 17 23 19 13 7 3 9 3 3 5 3 3 ],[0.98 0.96 0.92]);
      | plot([0 0 55 55 0 ],[0 26 26 0 0 ]);
      | fprintf('','COMMENT: end icon graphics');
      | fprintf('','COMMENT: begin icon text');
      | color('black');port_label('output',1,'0');
      | fprintf('','COMMENT: end icon text');
      mask prompts: arith_type_sgadvanced ""; arith_type "Type"; const "Constant value"; n_bits "Number of bits"; bin_pt "Binary point"; explicit_period_sgadvanced ""; explicit_period "Sampled constant"; period "Sample period"; dsp48_infoedit ""; equ "DSP48 operation"; opselect_sgadvanced ""; opselect "Operation select"; inp2_sgadvanced ""; inp2 "Z mux"; opr_sgadvanced ""; opr "Operand"; inp1_sgadvanced ""; inp1 "YX muxes"; carry_sgadvanced ""; carry "Carry input"; dbl_ovrd_sgadvanced ""; dbl_ovrd "Override with doubles"; has_advanced_control ""; sggui_pos ""; block_type ""; block_version ""; sg_icon_stat ""; sg_mask_display ""; sg_list_contents ""; sg_blockgui_xml ""
      mask help: Xilinx Constant Block
      mask init: same as warplab_mimo_4x4/CaptureDone/zero3
      settings: CopyFcn=xlBlockMoveCallback(gcbh);  DeleteFcn=xlDestroyGui(gcbh);  ModelCloseFcn=xlDestroyGui(gcbh);  PreSaveFcn=xlBlockPreSaveCallback(gcbh);  PostSaveFcn=xlBlockPostSaveCallback(gcbh);  DestroyFcn=xlDestroyGui(gcbh);  OpenFcn=xlOpenGui(gcbh, 'constant_gui.xml', @constantenablement, @constantaction)  CloseFcn=xlDestroyGui(gcbh);  MoveFcn=xlBlockMoveCallback(gcbh);
      mask Help: eval('xlWeb(xlhtmldoclink(''Constant''))');
      mask StyleString: edit,popup(Boolean|Signed (2's comp)|Unsigned|DSP48 Instruction),edit,edit,edit,edit,checkbox,edit,edit,edit,edit,popup(C + A*B|PCIN + A*B|P + A*B|A * B|C + A:B|C - A:B|C|Custom),edit,popup(0|PCIN|P|C|PCIN>>17|P>>17),edit,popup(+|-),edit,popup(0|P|A:B|A*B|C|P+C|A:B+C),edit,popup(0|1|CIN|~SIGN(P or PCIN)|~SIGN(A*B or A:B)|~SIGND(A*B or A:B)),edit,checkbox,edit,edit,edit,edit,edit,edit,edit,edit
      mask Display:
      | fprintf('','COMMENT: begin icon graphics');
      | patch([0 55 55 0 ],[0 0 26 26 ],[0.77 0.82 0.91]);
      | patch([20 16 22 16 20 27 29 31 38 32 26 22 28 22 26 32 38 31 29 27 20 ],[3 7 13 19 23 23 21 23 23 17 23 19 13 7 3 9 3 3 5 3 3 ],[0.98 0.96 0.92]);
      | plot([0 0 55 55 0 ],[0 26 26 0 0 ]);
      | fprintf('','COMMENT: end icon graphics');
      | fprintf('','COMMENT: begin icon text');
      | color('black');port_label('output',1,'0');
      | fprintf('','COMMENT: end icon text');
  zero1 : S-Function  LoadFcn=xlBlockLoadCallback(gcbh);  FunctionName=sysgen  Parameters=ptable_  mask(Xilinx Constant Block Block){arith_type_sgadvanced=, arith_type=Unsigned, const=0, n_bits=1, bin_pt=0, explicit_period_sgadvanced=, explicit_period=off, period=1, dsp48_infoedit=The use of this block for DSP48 instructions is deprecated.  Please use the Opmode block., equ=P=C, opselect_sgadvanced=, opselect=C, inp2_sgadvanced=, inp2=PCIN>>17, opr_sgadvanced=, opr=+, inp1_sgadvanced=, inp1=P, carry_sgadvanced=, carry=CIN, dbl_ovrd_sgadvanced=, dbl_ovrd=off, has_advanced_control=0, sggui_pos=-1,-1,-1,-1, block_type=constant, block_version=VER_STRING_GOES_HERE, sg_icon_stat=20,18,0,1,white,blue,0,c7c04a0c, sg_mask_display=|, sg_list_contents=, sg_blockgui_xml=}
      mask sg_mask_display=|
      | fprintf('','COMMENT: begin icon graphics');
      | patch([0 55 55 0 ],[0 0 26 26 ],[0.77 0.82 0.91]);
      | patch([20 16 22 16 20 27 29 31 38 32 26 22 28 22 26 32 38 31 29 27 20 ],[3 7 13 19 23 23 21 23 23 17 23 19 13 7 3 9 3 3 5 3 3 ],[0.98 0.96 0.92]);
      | plot([0 0 55 55 0 ],[0 26 26 0 0 ]);
      | fprintf('','COMMENT: end icon graphics');
      | fprintf('','COMMENT: begin icon text');
      | color('black');port_label('output',1,'0');
      | fprintf('','COMMENT: end icon text');
      mask prompts: arith_type_sgadvanced ""; arith_type "Type"; const "Constant value"; n_bits "Number of bits"; bin_pt "Binary point"; explicit_period_sgadvanced ""; explicit_period "Sampled constant"; period "Sample period"; dsp48_infoedit ""; equ "DSP48 operation"; opselect_sgadvanced ""; opselect "Operation select"; inp2_sgadvanced ""; inp2 "Z mux"; opr_sgadvanced ""; opr "Operand"; inp1_sgadvanced ""; inp1 "YX muxes"; carry_sgadvanced ""; carry "Carry input"; dbl_ovrd_sgadvanced ""; dbl_ovrd "Override with doubles"; has_advanced_control ""; sggui_pos ""; block_type ""; block_version ""; sg_icon_stat ""; sg_mask_display ""; sg_list_contents ""; sg_blockgui_xml ""
      mask help: Xilinx Constant Block
      mask init: same as warplab_mimo_4x4/CaptureDone/zero3
      settings: CopyFcn=xlBlockMoveCallback(gcbh);  DeleteFcn=xlDestroyGui(gcbh);  ModelCloseFcn=xlDestroyGui(gcbh);  PreSaveFcn=xlBlockPreSaveCallback(gcbh);  PostSaveFcn=xlBlockPostSaveCallback(gcbh);  DestroyFcn=xlDestroyGui(gcbh);  OpenFcn=xlOpenGui(gcbh, 'constant_gui.xml', @constantenablement, @constantaction)  CloseFcn=xlDestroyGui(gcbh);  MoveFcn=xlBlockMoveCallback(gcbh);
      mask Help: eval('xlWeb(xlhtmldoclink(''Constant''))');
      mask StyleString: edit,popup(Boolean|Signed (2's comp)|Unsigned|DSP48 Instruction),edit,edit,edit,edit,checkbox,edit,edit,edit,edit,popup(C + A*B|PCIN + A*B|P + A*B|A * B|C + A:B|C - A:B|C|Custom),edit,popup(0|PCIN|P|C|PCIN>>17|P>>17),edit,popup(+|-),edit,popup(0|P|A:B|A*B|C|P+C|A:B+C),edit,popup(0|1|CIN|~SIGN(P or PCIN)|~SIGN(A*B or A:B)|~SIGND(A*B or A:B)),edit,checkbox,edit,edit,edit,edit,edit,edit,edit,edit
      mask Display:
      | fprintf('','COMMENT: begin icon graphics');
      | patch([0 55 55 0 ],[0 0 26 26 ],[0.77 0.82 0.91]);
      | patch([20 16 22 16 20 27 29 31 38 32 26 22 28 22 26 32 38 31 29 27 20 ],[3 7 13 19 23 23 21 23 23 17 23 19 13 7 3 9 3 3 5 3 3 ],[0.98 0.96 0.92]);
      | plot([0 0 55 55 0 ],[0 26 26 0 0 ]);
      | fprintf('','COMMENT: end icon graphics');
      | fprintf('','COMMENT: begin icon text');
      | color('black');port_label('output',1,'0');
      | fprintf('','COMMENT: end icon text');
  32b : Outport
  wires:
  zero/1 -> Concat1/1
  Concat1/1 -> Concat3/2
  zero1/1 -> Concat2/1
  Concat2/1 -> Concat4/2
  Concat4/1 -> Concat5/1
  Concat3/1 -> Concat5/2
  OTR_I/1 -> Concat4/1
  Concat5/1 -> 32b/1
  ADC_I/1 -> Reinterpret/1
  OTR_Q/1 -> Concat3/1
  ADC_Q/1 -> Reinterpret1/1
  Reinterpret/1 -> Concat2/2
  Reinterpret1/1 -> Concat1/2

== system warplab_mimo_4x4/Radio_3_Outputs/Radio_3_DAC_I ==
  I : Inport
  Convert : S-Function  LoadFcn=xlBlockLoadCallback(gcbh);  FunctionName=sysgen  Parameters=ptable_  mask(Xilinx Type Converter Block){infoedit=Hardware notes: rounding and saturating require hardware resources; truncating and wrapping do not., arith_type_sgadvanced=, arith_type=Signed  (2's comp), n_bits=16, bin_pt=15, quantization_sgadvanced=, quantization=Truncate, overflow_sgadvanced=, overflow=Flag as error, latency=0, dbl_ovrd_sgadvanced=, dbl_ovrd=off, pipeline_sgadvanced=, pipeline=off, xl_use_area_sgadvanced=, xl_use_area=off, xl_area=[0,0,0,0,0,0,0], has_advanced_control=0, sggui_pos=20,20,374,366, block_type=convert, block_version=VER_STRING_GOES_HERE, sg_icon_stat=45,20,1,1,white,blue,0,0eb6e735, sg_mask_display=|, sg_list_contents=, sg_blockgui_xml=}
      mask sg_mask_display=|
      | fprintf('','COMMENT: begin icon graphics ');
      | patch([0 45 45 0 ],[0 0 20 20 ],[0.77 0.82 0.91]);
      | patch([17 14 19 14 17 22 23 24 30 26 22 19 24 19 22 26 30 24 23 22 17 ],[2 5 10 15 18 18 17 18 18 14 18 15 10 5 2 6 2 2 3 2 2 ],[0.98 0.96 0.92]);
      | plot([0 0 45 45 0 ],[0 20 20 0 0 ]);
      | fprintf('','COMMENT: end icon graphics');
      |
      | fprintf('','COMMENT: begin icon text ');
      | color('black');port_label('output',1,'cast');
      | fprintf('','COMMENT: end icon text');
      mask prompts: infoedit ""; arith_type_sgadvanced ""; arith_type "Type"; n_bits "Number of bits"; bin_pt "Binary point"; quantization_sgadvanced ""; overflow_sgadvanced ""; dbl_ovrd_sgadvanced ""; dbl_ovrd "Override with doubles"; pipeline_sgadvanced ""; pipeline "Pipeline for maximum performance"; xl_use_area_sgadvanced ""; xl_use_area "Define FPGA area for resource estimation"; xl_area "FPGA area [slices, FFs, BRAMs, LUTs, IOBs, emb. mults, TBUFs]"; has_advanced_control ""; sggui_pos ""; block_type ""; block_version ""; sg_icon_stat ""; sg_mask_display ""; sg_list_contents ""; sg_blockgui_xml ""
      mask help: Hardware notes: rounding and saturating require hardware resources; truncating and wrapping do not.
      mask init: same as warplab_mimo_4x4/Mem_Control/Convert1
      settings: CopyFcn=xlBlockMoveCallback(gcbh);  DeleteFcn=xlDestroyGui(gcbh);  ModelCloseFcn=xlDestroyGui(gcbh);  PreSaveFcn=xlBlockPreSaveCallback(gcbh);  PostSaveFcn=xlBlockPostSaveCallback(gcbh);  DestroyFcn=xlDestroyGui(gcbh);  OpenFcn=xlOpenGui(gcbh, 'convert_gui.xml', @convertenablement, -1)  CloseFcn=xlDestroyGui(gcbh);  MoveFcn=xlBlockMoveCallback(gcbh);
      mask Help: eval('xlWeb(xlhtmldoclink(''Convert''))');
      mask StyleString: edit,edit,popup(Boolean|Signed  (2's comp)|Unsigned),edit,edit,edit,popup(Truncate|Round  (unbiased: +/- Inf)|Round  (unbiased: Even Values)),edit,popup(Wrap|Saturate|Flag as error),edit,edit,checkbox,edit,checkbox,edit,checkbox,edit,edit,edit,edit,edit,edit,edit,edit,edit
      mask Display:
      | fprintf('','COMMENT: begin icon graphics ');
      | patch([0 45 45 0 ],[0 0 20 20 ],[0.77 0.82 0.91]);
      | patch([17 14 19 14 17 22 23 24 30 26 22 19 24 19 22 26 30 24 23 22 17 ],[2 5 10 15 18 18 17 18 18 14 18 15 10 5 2 6 2 2 3 2 2 ],[0.98 0.96 0.92]);
      | plot([0 0 45 45 0 ],[0 20 20 0 0 ]);
      | fprintf('','COMMENT: end icon graphics');
      | 
      | fprintf('','COMMENT: begin icon text ');
      | color('black');port_label('output',1,'cast');
      | fprintf('','COMMENT: end icon text');
  radio3_DAC_I : S-Function  LoadFcn=xlBlockLoadCallback(gcbh);  FunctionName=sysgen  Parameters=ptable_  mask(Xilinx Gateway Out Block){infoedit=Gateway out block.  Converts Xilinx fixed point inputs into ouputs of type Simulink integer, double, or fixed point.<P><P>Hardware notes:  In hardware these blocks become top level output ports or are discarded, depending on how they are configured., hdl_port_sgadvanced=, hdl_port=on, timing_constraint_sgadvanced=, timing_constraint=None, locs_specified_sgadvanced=, locs_specified=off, LOCs={}, xl_use_area_sgadvanced=, xl_use_area=off, xl_area=[0,0,0,0,0,0,0], sginterface=, has_advanced_control=0, sggui_pos=-1,-1,-1,-1, block_type=gatewayout, block_version=VER_STRING_GOES_HERE, sg_icon_stat=55,22,1,1,white,yellow,0,f0cec300, sg_mask_display=|, sg_list_contents=, sg_blockgui_xml=}
      mask sg_mask_display=|
      | fprintf('','COMMENT: begin icon graphics ');
      | patch([0 55 55 0 ],[0 0 22 22 ],[0.95 0.93 0.65]);
      | patch([22 18 23 18 22 28 30 32 38 33 28 25 31 25 28 33 38 32 30 28 22 ],[2 6 11 16 20 20 18 20 20 15 20 17 11 5 2 7 2 2 4 2 2 ],[0.98 0.96 0.92]);
      | plot([0 0 55 55 0 ],[0 22 22 0 0 ]);
      | fprintf('','COMMENT: end icon graphics');
      |
      | fprintf('','COMMENT: begin icon text ');
      | color('black');port_label('input',1,' ');
      | color('black');port_label('output',1,'\fontsize{11pt}\bf Out ','texmode','on');
      | fprintf('','COMMENT: end icon text');
      | fprintf('','COMMENT: Make no changes above this line -- machine generated code. ');
      mask prompts: infoedit ""; hdl_port_sgadvanced ""; hdl_port "Translate into output port"; timing_constraint_sgadvanced ""; timing_constraint "IOB timing constraint"; locs_specified_sgadvanced ""; locs_specified "Specify IOB location constraints"; LOCs "IOB pad locations (cell array {'MSB', ..., 'LSB'})"; xl_use_area_sgadvanced ""; xl_use_area "Define FPGA area for resource estimation"; xl_area "FPGA area [slices, FFs, BRAMs, LUTs, IOBs, emb. mults, TBUFs]"; sginterface ""; has_advanced_control ""; sggui_pos ""; block_type ""; block_version ""; sg_icon_stat ""; sg_mask_display ""; sg_list_contents ""; sg_blockgui_xml ""
      mask help:
      | Gateway out block.  Converts Xilinx fixed point inputs into ouputs of type Simulink integer, double, or fixed point.
      |
      | Hardware notes:  In hardware these blocks become top level output ports or are discarded, depending on how they are configured.
      mask init: same as warplab_mimo_4x4/RSSI_ADC_CLK
      settings: CopyFcn=xlBlockMoveCallback(gcbh);  DeleteFcn=xlDestroyGui(gcbh);  ModelCloseFcn=xlDestroyGui(gcbh);  PreSaveFcn=xlBlockPreSaveCallback(gcbh);  PostSaveFcn=xlBlockPostSaveCallback(gcbh);  DestroyFcn=xlDestroyGui(gcbh);  OpenFcn=xlOpenGui(gcbh, 'gatewayout_gui.xml', @gatewayoutenablement, -1)  CloseFcn=xlDestroyGui(gcbh);  MoveFcn=xlBlockMoveCallback(gcbh);
      mask Help: eval('xlWeb(xlhtmldoclink(''Gateway Out''))');
      mask StyleString: edit,edit,checkbox,edit,popup(None|Data Rate|Data Rate;  Set 'FAST' Attribute),edit,checkbox,edit,edit,checkbox,edit,edit,edit,edit,edit,edit,edit,edit,edit,edit
      mask Display:
      | fprintf('','COMMENT: begin icon graphics ');
      | patch([0 55 55 0 ],[0 0 22 22 ],[0.95 0.93 0.65]);
      | patch([22 18 23 18 22 28 30 32 38 33 28 25 31 25 28 33 38 32 30 28 22 ],[2 6 11 16 20 20 18 20 20 15 20 17 11 5 2 7 2 2 4 2 2 ],[0.98 0.96 0.92]);
      | plot([0 0 55 55 0 ],[0 22 22 0 0 ]);
      | fprintf('','COMMENT: end icon graphics');
      | 
      | fprintf('','COMMENT: begin icon text ');
      | color('black');port_label('input',1,' ');
      | color('black');port_label('output',1,'\fontsize{11pt}\bf Out ','texmode','on');
      | fprintf('','COMMENT: end icon text');
      | fprintf('','COMMENT: Make no changes above this line -- machine generated code. ');
  I_out : Outport
  wires:
  radio3_DAC_I/1 -> I_out/1
  I/1 -> Convert/1
  Convert/1 -> radio3_DAC_I/1
